simulink model "ILC_keitaro"  (R2019a)
settings: Solver=VariableStepAuto  StartTime=0.0  StopTime=10  RelTol=1e-3
values from neighbouring files (symbols this model uses):
  K = 10    [ilc_halp.m]
libraries: cstblocks x1
settings Model: Creator=capn  LastModifiedBy=keimu
settings DataIOCC: ReturnWorkspaceOutputs=off
settings DebuggingCC: ArithmeticOperatorsInVariantConditions=warning
settings SFSimCC: SimUseLocalCustomCode=off
settings RTWCC: RTWUseLocalCustomCode=off
settings CodeAppCC: StateflowObjectComments=on

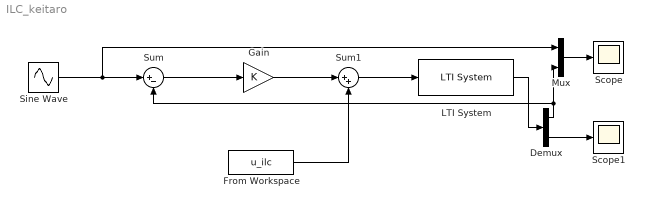
== system ILC_keitaro ==
  Demux : Demux  Outputs=2
  From Workspace : FromWorkspace  VariableName=u_ilc  SampleTime=0
  Gain : Gain  Gain=K
  LTI System : cstblocks/LTI System  sys=Pd  IC=[]
  Mux : Mux  Inputs=2
  Scope : Scope
  Scope1 : Scope
  Sine Wave : Sin  Frequency=6.2831853  SampleTime=0
  Sum : Sum  Inputs=|+-
  Sum1 : Sum  Inputs=|++
  wires:
  Sum/1 -> Gain/1
  Gain/1 -> Sum1/1
  Sum1/1 -> LTI System/1
  Sine Wave/1 -> Mux/1, Sum/1
  From Workspace/1 -> Sum1/2
  Mux/1 -> Scope/1
  LTI System/1 -> Demux/1
  Demux/1 -> Sum/2, Mux/2
  Demux/2 -> Scope1/1
